simulink model "smROB2"  (R2022b)
settings: Solver=VariableStepAuto  StartTime=0.0  StopTime=100  FixedStep=1  RelTol=1e-3
values from neighbouring files (symbols this model uses):
  B1 = 2    [ROB2.m]
  B2 = 2    [ROB2.m]
  g = 9.81    [ROB2.m]
  l1 = 1    [ROB2.m]
  l2 = 1    [ROB2.m]
  m1 = 5    [ROB2.m]
  m2 = 59    [ROB2.m]
libraries: slpidlib x2
settings Model: Creator=ASUS TUF  LastModifiedBy=ASUS TUF
settings DebuggingCC: AlgebraicLoopMsg=none

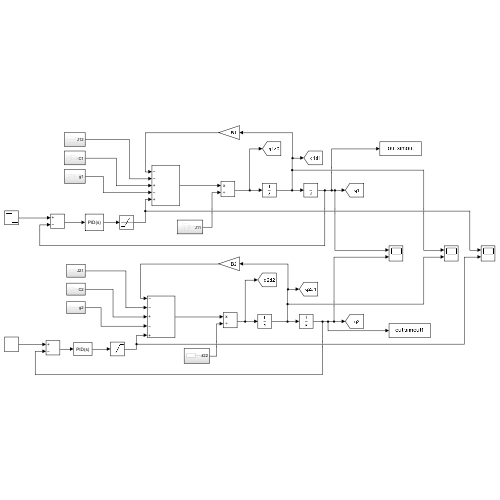
[thumbnail: Simulink's stored preview of the top-level diagram]
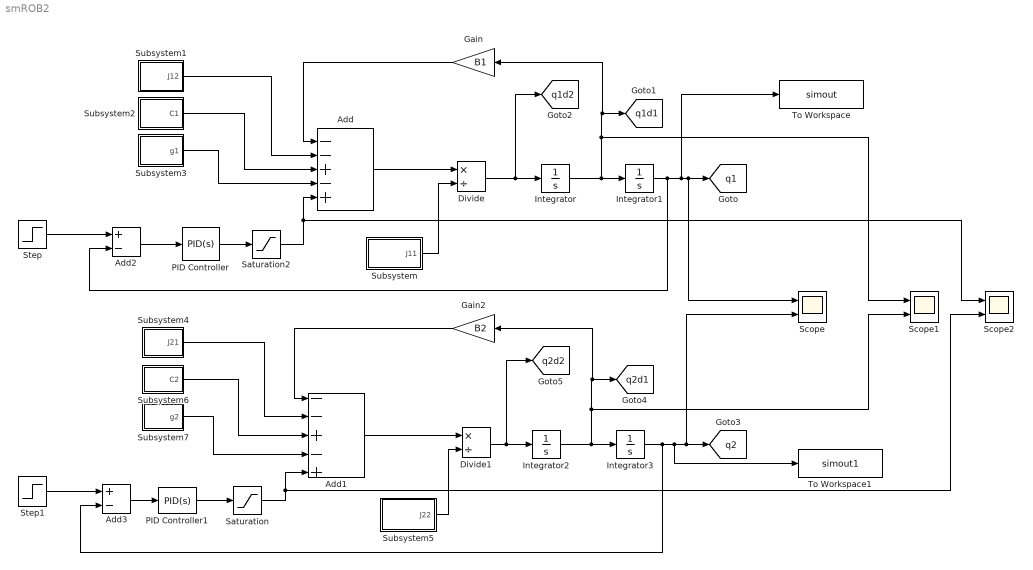
== system smROB2 ==
  Add : Sum  Inputs=--+-+
  Add1 : Sum  Inputs=--+-+
  Add2 : Sum  Inputs=+-
  Add3 : Sum  Inputs=+-
  Divide : Product  Inputs=*/  RndMeth=Zero  SaturateOnIntegerOverflow=on
  Divide1 : Product  Inputs=*/  RndMeth=Zero  SaturateOnIntegerOverflow=on
  Gain : Gain  Gain=B1
  Gain2 : Gain  Gain=B2
  Integrator{,1..3} (4 alike) : Integrator
  PID Controller : slpidlib/PID Controller  Controller=PID  Form=Parallel  TimeDomain=Continuous-time  UseExternalTs=off  SampleTime=-1  IntegratorMethod=Forward Euler  FilterMethod=Forward Euler  ControllerParametersSource=internal  P=500  I=50  UseKiTs=off  D=1500  N=100  UseFilter=on  TunerSelectOption=Transfer Function Based (PID Tuner App)  InitialConditionSource=internal  InitialConditionForIntegrator=0  InitialConditionForFilter=0  DifferentiatorICPrevScaledInput=0  ExternalReset=none  TrackingMode=off  Kt=1  LimitOutput=off  SatLimitsSource=internal  UpperSaturationLimit=inf  LowerSaturationLimit=-inf  LinearizeAsGain=on  AntiWindupMode=none  Kb=1  LimitIntegrator=off  UpperIntegratorSaturationLimit=inf  LowerIntegratorSaturationLimit=-inf  POutMin=[]  POutMax=[]  IOutMin=[]  IOutMax=[]  DOutMin=[]  DOutMax=[]  NOutMin=[]  NOutMax=[]  SumOutMin=[]  SumOutMax=[]  SaturationOutMin=[]  SaturationOutMax=[]  PParamMin=[]  PParamMax=[]  IParamMin=[]  IParamMax=[]  DParamMin=[]  DParamMax=[]  NParamMin=[]  NParamMax=[]  KbParamMin=[]  KbParamMax=[]  KtParamMin=[]  KtParamMax=[]  KbOutMin=[]  KbOutMax=[]  KtOutMin=[]  KtOutMax=[]  IntegratorOutMin=[]  IntegratorOutMax=[]  FilterOutMin=[]  FilterOutMax=[]  SumI1OutMin=[]  SumI1OutMax=[]  SumI2OutMin=[]  SumI2OutMax=[]  SumI3OutMin=[]  SumI3OutMax=[]  SumI4OutMin=[]  SumI4OutMax=[]  SumDOutMin=[]  SumDOutMax=[]  DifferentiatorOutMin=[]  DifferentiatorOutMax=[]  FilterDiffOutCoefMin=[]  FilterDiffOutCoefMax=[]  ReciprocalOutMin=[]  ReciprocalOutMax=[]  SumDenOutMin=[]  SumDenOutMax=[]  SumNumOutMin=[]  SumNumOutMax=[]  DivideOutMin=[]  DivideOutMax=[]  UdiffTsProdOutMin=[]  UdiffTsProdOutMax=[]  NTsProdOutMin=[]  NTsProdOutMax=[]  UintegralTsProdOutMin=[]  UintegralTsProdOutMax=[]  UngainTsProdOutMin=[]  UngainTsProdOutMax=[]  ClampingZeroOutDataTypeStr=Inherit: Inherit via back propagation  ClampingZeroOutMin=[]  ClampingZeroOutMax=[]  FilterDenConstantOutDataTypeStr=Inherit: Inherit via back propagation  FilterDenConstantOutMin=[]  FilterDenConstantOutMax=[]  PCopyOutDataTypeStr=Inherit: Inherit via back propagation  PCopyOutMin=[]  PCopyOutMax=[]  NCopyOutDataTypeStr=Inherit: Inherit via back propagation  NCopyOutMin=[]  NCopyOutMax=[]  IntegratorContinuousStateAttributes=''  IntegratorStateMustResolveToSignalObject=off  IntegratorRTWStateStorageClass=Auto  FilterContinuousStateAttributes=''  FilterStateMustResolveToSignalObject=off  FilterRTWStateStorageClass=Auto  ParallelPVariant=InternalParameters  IdealPVariant=Disabled  IVariant=InternalParameters  DVariant=InternalParameters  IntegratorVariant=Continuous  SatVariant=Disabled  AWVariant=Passthrough  PCopyVariant=Disabled  TRVariant=Disabled  FdbkBlocksVariant=Forward  IdealPFdbkVariant=Disabled  SatFdbkVariant=Disabled  DerivativeFilterVariant=ContFilter  NVariant=InternalParameters  NCopyVariant=Disabled  FilterICVariant=InternalICsFilter  IntegratorICVariant=InternalICs  ExternalResetVariant=Disabled  TRSumVariant=Passthrough  SumFdbkVariant=Disabled  SumVariant=Sum_PID  TsampFilterVariant=InternalTs  TsampNgainVariant=Passthrough  TsampIntegralVariant=Passthrough  ExternalSaturationOutDataTypeStr=Inherit: Same as second input
  PID Controller1 : slpidlib/PID Controller  Controller=PID  Form=Parallel  TimeDomain=Continuous-time  UseExternalTs=off  SampleTime=-1  IntegratorMethod=Forward Euler  FilterMethod=Forward Euler  ControllerParametersSource=internal  P=2700  I=50  UseKiTs=off  D=1500  N=100  UseFilter=on  TunerSelectOption=Transfer Function Based (PID Tuner App)  InitialConditionSource=internal  InitialConditionForIntegrator=0  InitialConditionForFilter=0  DifferentiatorICPrevScaledInput=0  ExternalReset=none  TrackingMode=off  Kt=1  LimitOutput=off  SatLimitsSource=internal  UpperSaturationLimit=inf  LowerSaturationLimit=-inf  LinearizeAsGain=off  AntiWindupMode=none  Kb=1  LimitIntegrator=off  UpperIntegratorSaturationLimit=100  LowerIntegratorSaturationLimit=-100  RndMeth=Zero  POutMin=[]  POutMax=[]  IOutMin=[]  IOutMax=[]  DOutMin=[]  DOutMax=[]  NOutMin=[]  NOutMax=[]  SumOutMin=[]  SumOutMax=[]  SaturationOutMin=[]  SaturationOutMax=[]  PParamMin=[]  PParamMax=[]  IParamMin=[]  IParamMax=[]  DParamMin=[]  DParamMax=[]  NParamMin=[]  NParamMax=[]  KbParamMin=[]  KbParamMax=[]  KtParamMin=[]  KtParamMax=[]  KbOutMin=[]  KbOutMax=[]  KtOutMin=[]  KtOutMax=[]  IntegratorOutMin=[]  IntegratorOutMax=[]  FilterOutMin=[]  FilterOutMax=[]  SumI1OutMin=[]  SumI1OutMax=[]  SumI2OutMin=[]  SumI2OutMax=[]  SumI3OutMin=[]  SumI3OutMax=[]  SumI4OutMin=[]  SumI4OutMax=[]  SumDOutMin=[]  SumDOutMax=[]  DifferentiatorOutMin=[]  DifferentiatorOutMax=[]  FilterDiffOutCoefMin=[]  FilterDiffOutCoefMax=[]  ReciprocalOutMin=[]  ReciprocalOutMax=[]  SumDenOutMin=[]  SumDenOutMax=[]  SumNumOutMin=[]  SumNumOutMax=[]  DivideOutMin=[]  DivideOutMax=[]  UdiffTsProdOutMin=[]  UdiffTsProdOutMax=[]  NTsProdOutMin=[]  NTsProdOutMax=[]  UintegralTsProdOutMin=[]  UintegralTsProdOutMax=[]  UngainTsProdOutMin=[]  UngainTsProdOutMax=[]  ClampingZeroOutDataTypeStr=Inherit: Inherit via back propagation  ClampingZeroOutMin=[]  ClampingZeroOutMax=[]  FilterDenConstantOutDataTypeStr=Inherit: Inherit via back propagation  FilterDenConstantOutMin=[]  FilterDenConstantOutMax=[]  PCopyOutDataTypeStr=Inherit: Inherit via back propagation  PCopyOutMin=[]  PCopyOutMax=[]  NCopyOutDataTypeStr=Inherit: Inherit via back propagation  NCopyOutMin=[]  NCopyOutMax=[]  IntegratorContinuousStateAttributes=''  IntegratorStateMustResolveToSignalObject=off  IntegratorRTWStateStorageClass=Auto  FilterContinuousStateAttributes=''  FilterStateMustResolveToSignalObject=off  FilterRTWStateStorageClass=Auto  ParallelPVariant=InternalParameters  IdealPVariant=Disabled  IVariant=InternalParameters  DVariant=InternalParameters  IntegratorVariant=Continuous  SatVariant=Disabled  AWVariant=Passthrough  PCopyVariant=Disabled  TRVariant=Disabled  FdbkBlocksVariant=Forward  IdealPFdbkVariant=Disabled  SatFdbkVariant=Disabled  DerivativeFilterVariant=ContFilter  NVariant=InternalParameters  NCopyVariant=Disabled  FilterICVariant=InternalICsFilter  IntegratorICVariant=InternalICs  ExternalResetVariant=Disabled  TRSumVariant=Passthrough  SumFdbkVariant=Disabled  SumVariant=Sum_PID  TsampFilterVariant=InternalTs  TsampNgainVariant=Passthrough  TsampIntegralVariant=Passthrough  ExternalSaturationOutDataTypeStr=Inherit: Same as second input
  Saturation : Saturate  UpperLimit=374  LowerLimit=-374
  Saturation2 : Saturate  UpperLimit=374  LowerLimit=-374
  Scope : Scope  NumInputPorts=2
  Scope1 : Scope  NumInputPorts=2
  Scope2 : Scope  NumInputPorts=2
  Step : Step  Time=0  After=-pi/2  SampleTime=0
  Step1 : Step  Time=0  Before=1  After=-pi/4  SampleTime=0
  Subsystem : Subsystem
  Subsystem1 : Subsystem
  Subsystem2 : Subsystem
  Subsystem3 : Subsystem
  Subsystem4 : Subsystem
  Subsystem5 : Subsystem
  Subsystem6 : Subsystem
  Subsystem7 : Subsystem
  To Workspace : ToWorkspace  VariableName=simout  SaveFormat=Timeseries  SampleTime=-1
  To Workspace1 : ToWorkspace  VariableName=simout1  SaveFormat=Timeseries  SampleTime=-1
  tag scope: q1=global, q1d1=global, q1d2=global, q2=global, q2d1=global, q2d2=global
  wires:
  Add/1 -> Divide/1
  Divide/1 -> [q1d2], Integrator/1
  Integrator/1 -> Scope1/1, Gain/1, [q1d1], Integrator1/1
  Gain/1 -> Add/1
  Divide1/1 -> [q2d2], Integrator2/1
  Gain2/1 -> Add1/1
  Integrator2/1 -> Gain2/1, [q2d1], Scope1/2, Integrator3/1
  Subsystem/1(J11) -> Divide/2
  Subsystem2/1(C1) -> Add/3
  Integrator1/1 -> To Workspace/1, Scope/1, [q1], Add2/2
  Subsystem1/1(J12) -> Add/2
  Subsystem3/1(g1) -> Add/4
  Subsystem4/1(J21) -> Add1/2
  Subsystem6/1(C2) -> Add1/3
  Subsystem7/1(g2) -> Add1/4
  Add1/1 -> Divide1/1
  Integrator3/1 -> Add3/2, To Workspace1/1, Scope/2, [q2]
  Subsystem5/1(J22) -> Divide1/2
  Step1/1 -> Add3/1
  Step/1 -> Add2/1
  Add2/1 -> PID Controller/1
  Add3/1 -> PID Controller1/1
  PID Controller1/1 -> Saturation/1
  PID Controller/1 -> Saturation2/1
  Saturation2/1 -> Scope2/1, Add/5
  Saturation/1 -> Add1/5, Scope2/2

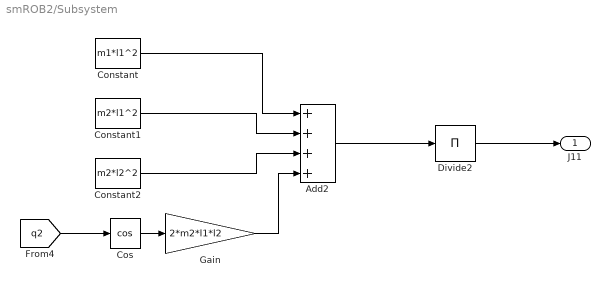
== system smROB2/Subsystem ==
  Add2 : Sum  Inputs=++++
  Constant : Constant  Value=m1*l1^2
  Constant1 : Constant  Value=m2*l1^2
  Constant2 : Constant  Value=m2*l2^2
  Cos : Trigonometry  Operator=cos
  Divide2 : Product  Inputs=*  RndMeth=Zero  SaturateOnIntegerOverflow=on
  Gain : Gain  Gain=2*m2*l1*l2
  J11 : Outport
  wires:
  Constant2/1 -> Add2/3
  [q2] -> Cos/1
  Constant/1 -> Add2/1
  Constant1/1 -> Add2/2
  Cos/1 -> Gain/1
  Add2/1 -> Divide2/1
  Gain/1 -> Add2/4
  Divide2/1 -> J11/1

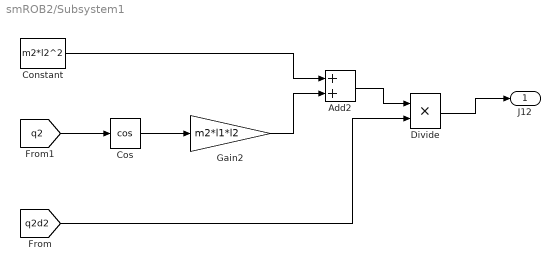
== system smROB2/Subsystem1 ==
  Add2 : Sum
  Constant : Constant  Value=m2*l2^2
  Cos : Trigonometry  Operator=cos
  Divide : Product  Inputs=**  RndMeth=Zero  SaturateOnIntegerOverflow=on
  Gain2 : Gain  Gain=m2*l1*l2
  J12 : Outport
  wires:
  [q2] -> Cos/1
  Constant/1 -> Add2/1
  Cos/1 -> Gain2/1
  Gain2/1 -> Add2/2
  Divide/1 -> J12/1
  Add2/1 -> Divide/1
  [q2d2] -> Divide/2

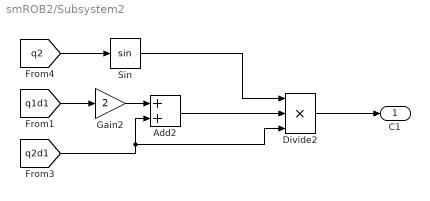
== system smROB2/Subsystem2 ==
  Add2 : Sum
  Divide2 : Product  Inputs=***  RndMeth=Zero  SaturateOnIntegerOverflow=on
  Gain2 : Gain  Gain=2
  Sin : Trigonometry
  C1 : Outport
  wires:
  [q2d1] -> Divide2/3, Add2/2
  Add2/1 -> Divide2/2
  [q2] -> Sin/1
  [q1d1] -> Gain2/1
  Sin/1 -> Divide2/1
  Divide2/1 -> C1/1
  Gain2/1 -> Add2/1

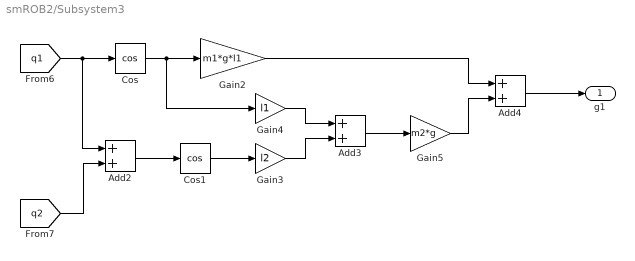
== system smROB2/Subsystem3 ==
  Add2 : Sum
  Add3 : Sum
  Add4 : Sum
  Cos : Trigonometry  Operator=cos
  Cos1 : Trigonometry  Operator=cos
  Gain2 : Gain  Gain=m1*g*l1
  Gain3 : Gain  Gain=l2
  Gain4 : Gain  Gain=l1
  Gain5 : Gain  Gain=m2*g
  g1 : Outport
  wires:
  Cos1/1 -> Gain3/1
  Add4/1 -> g1/1
  Add2/1 -> Cos1/1
  Cos/1 -> Gain4/1, Gain2/1
  Gain5/1 -> Add4/2
  [q1] -> Add2/1, Cos/1
  [q2] -> Add2/2
  Gain4/1 -> Add3/1
  Gain2/1 -> Add4/1
  Gain3/1 -> Add3/2
  Add3/1 -> Gain5/1

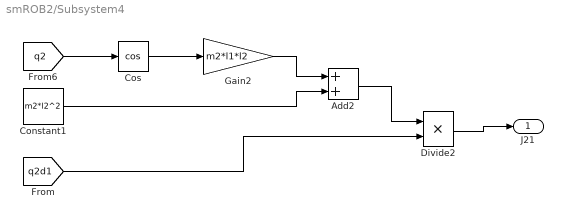
== system smROB2/Subsystem4 ==
  Add2 : Sum
  Constant1 : Constant  Value=m2*l2^2
  Cos : Trigonometry  Operator=cos
  Divide2 : Product  Inputs=**  RndMeth=Zero  SaturateOnIntegerOverflow=on
  Gain2 : Gain  Gain=m2*l1*l2
  J21 : Outport
  wires:
  Constant1/1 -> Add2/2
  Add2/1 -> Divide2/1
  Cos/1 -> Gain2/1
  Divide2/1 -> J21/1
  [q2] -> Cos/1
  Gain2/1 -> Add2/1
  [q2d1] -> Divide2/2

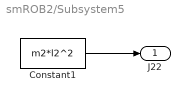
== system smROB2/Subsystem5 ==
  Constant1 : Constant  Value=m2*l2^2
  J22 : Outport
  wires:
  Constant1/1 -> J22/1

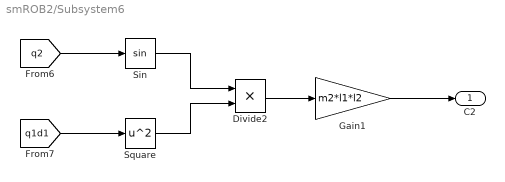
== system smROB2/Subsystem6 ==
  Divide2 : Product  Inputs=**  RndMeth=Zero  SaturateOnIntegerOverflow=on
  Gain1 : Gain  Gain=m2*l1*l2
  Sin : Trigonometry
  Square : Math  Operator=square
  C2 : Outport
  wires:
  Sin/1 -> Divide2/1
  [q2] -> Sin/1
  [q1d1] -> Square/1
  Square/1 -> Divide2/2
  Divide2/1 -> Gain1/1
  Gain1/1 -> C2/1

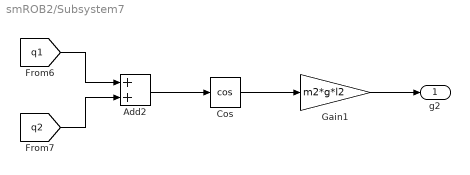
== system smROB2/Subsystem7 ==
  Add2 : Sum
  Cos : Trigonometry  Operator=cos
  Gain1 : Gain  Gain=m2*g*l2
  g2 : Outport
  wires:
  [q1] -> Add2/1
  Cos/1 -> Gain1/1
  Add2/1 -> Cos/1
  [q2] -> Add2/2
  Gain1/1 -> g2/1
